simulink model "abs_pci_stress"  (Simulink 8.0)
settings: Solver=ode1  SolverMode=SingleTasking  StartTime=0.0  StopTime=999999  FixedStep=0.01  RelTol=1e-3  AbsTol=1e-6
undefined symbols (not defined in the file): abspositionscale, abspowerscale, abstemperaturescale, absvelocityscale, RTDAC4PCIBaseAddress
libraries: simulink_extras x2, simulink x1
settings Model: Creator=jims  LastModifiedBy=inteco  SimulationMode=external  ExtModeTrigDuration=60000  BufferReuse=off
settings DataIOCC: ExternalInput=[]  InitialState=[]  LimitDataPoints=off  MaxDataPoints=5000  SignalLoggingSaveFormat=ModelDataLogs  SaveOutput=off  SaveTime=off  SignalLoggingName=sigsOut
settings OptimizationCC: BlockReduction=off  BooleanDataType=off  OptimizeBlockIOStorage=off  BufferReuse=off  ExpressionFolding=off  FoldNonRolledExpr=off  LocalBlockOutputs=off  InitFltsAndDblsToZero=on
settings DebuggingCC: SaveWithParameterizedLinksMsg=none  SignalResolutionControl=TryResolveAllWithWarning  SolverPrmCheckMsg=none  MultiTaskDSMMsg=warning  MultiTaskCondExecSysMsg=none  IntegerOverflowMsg=none  FcnCallInpInsideContextMsg=UseLocalSettings  StrictBusMsg=None
settings HardwareCC: ProdIntDivRoundTo=Zero  ProdEndianess=LittleEndian  ProdHWDeviceType=Generic->32-bit x86 compatible
settings RTWCC: SystemTargetFile=rtwin.tlc  TemplateMakefile=rtwin.tmf  Description=Real-Time Windows Target  ProcessScript=rtwin_make_rtw_hook  IncludeERTFirstTime=on  RTWCompilerOptimization=On
settings CodeAppCC: MaxIdLength=95
settings RTWinTargetCC: TargetLibSuffix=_rtwin.lib  TargetPreCompLibLocation=E:\apps_W64\MATLAB\x64_R2012b\toolbox\rtw\targets\rtwin\lib\win64  CodeReplacementLibrary=ANSI_C  RTWinDir=E:/apps_W64/MATLAB/X64_R2~1/toolbox/rtw/targets/rtwin  TargetArch=win64

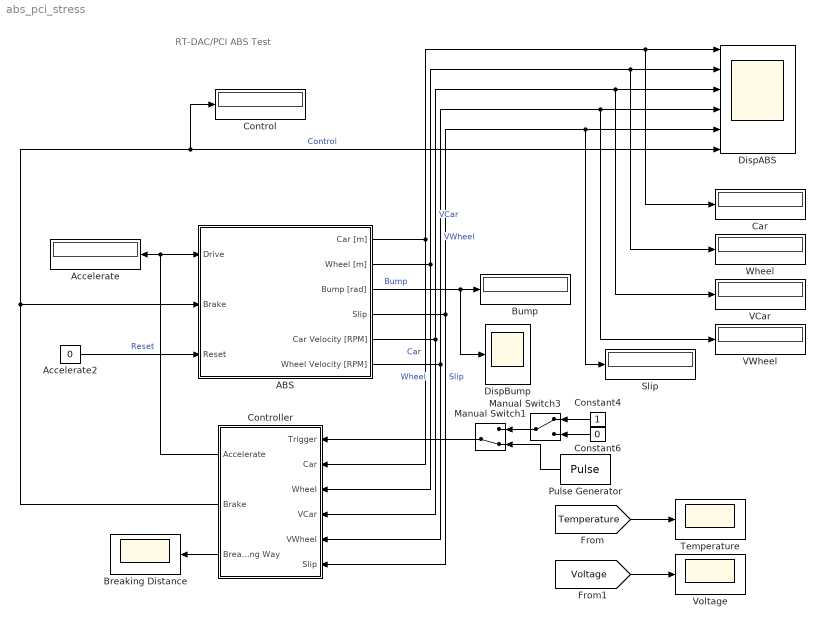
== system abs_pci_stress ==
  note: RT-DAC/PCI ABS Test
  ABS : Subsystem  mask{BaseAddress=RTDAC4PCIBaseAddress(-1,-1), T0=0.01}
      mask prompts: BaseAddress "Base Address"; T0 "Sample Time"
      mask Display: image(imread('abs.bmp'))
  Accelerate : Display
  Accelerate2 : Constant  Value=0
  Breaking Distance : Scope
      settings: TimeRange=2000  YMin=0  YMax=25  SaveName=BrakingDistance  MaxDataPoints=6000  Decimation=100
  Bump : Display
  Car : Display
  Constant4 : Constant
  Constant6 : Constant  Value=0
  Control : Display
  Controller : Subsystem
  DispABS : Scope  NumInputPorts=6
      settings: TimeRange=60  YMin=75~50~0~0~-0.4~0  YMax=250~225~1750~1750~1~1  SaveName=AbsHistory  MaxDataPoints=6000
  DispBump : Scope
      settings: TimeRange=60  YMin=3075  YMax=3275  SaveName=Vel  MaxDataPoints=6000
  Manual Switch1 : ManualSwitch  CurrentSetting=0
  Manual Switch3 : ManualSwitch
  Pulse Generator : DiscretePulseGenerator  PulseType=Time based  Period=15  PulseWidth=99
  Slip : Display
  Temperature : Scope
      settings: TimeRange=2000  YMin=20  YMax=28  SaveName=Temperature  MaxDataPoints=6000  Decimation=100
  VCar : Display
  VWheel : Display
  Voltage : Scope
      settings: TimeRange=60  YMin=18  YMax=28  SaveName=Temperature1  MaxDataPoints=6000
  Wheel : Display
  wires:
  ABS/4(Slip) -> Controller/6(Slip), DispABS/5, Slip/1  "Slip"
  ABS/6(Wheel Velocity [RPM]) -> Controller/5(VWheel), DispABS/4, VWheel/1  "VWheel"
  ABS/2(Wheel [m]) -> Controller/3(Wheel), DispABS/2, Wheel/1  "Wheel"
  ABS/1(Car [m]) -> Controller/2(Car), DispABS/1, Car/1  "Car"
  Controller/3(Breaking Way) -> Breaking Distance/1
  Constant6/1 -> Manual Switch3/2
  Constant4/1 -> Manual Switch3/1
  Controller/2(Brake) -> DispABS/6, Control/1, ABS/2(Brake)  "Control"
  ABS/5(Car Velocity [RPM]) -> Controller/4(VCar), DispABS/3, VCar/1  "VCar"
  Accelerate2/1 -> ABS/3(Reset)  "Reset"
  ABS/3(Bump [rad]) -> Bump/1, DispBump/1  "Bump"
  Controller/1(Accelerate) -> Accelerate/1, ABS/1(Drive)
  Manual Switch3/1 -> Manual Switch1/1
  Pulse Generator/1 -> Manual Switch1/2
  Manual Switch1/1 -> Controller/1(Trigger)
  [Temperature] -> Temperature/1
  [Voltage] -> Voltage/1

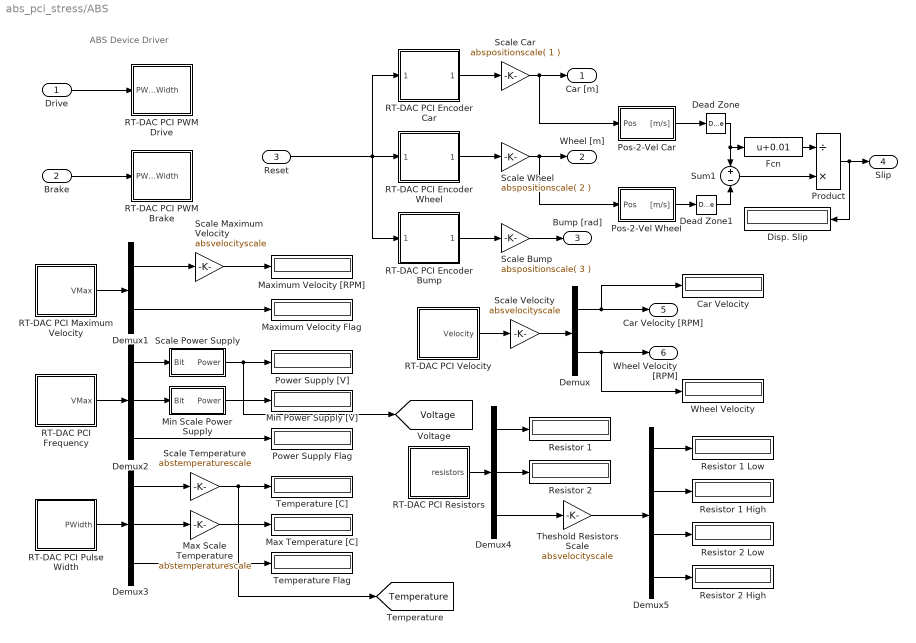
== system abs_pci_stress/ABS ==
  note: ABS Device Driver
  Drive : Inport
  Brake : Inport  Port=2
  Reset : Inport  Port=3
  Car Velocity : Display
  Dead Zone : DeadZone  LowerValue=-0.05  UpperValue=0.05  SaturateOnIntegerOverflow=on
  Dead Zone1 : DeadZone  LowerValue=-0.05  UpperValue=0.05  SaturateOnIntegerOverflow=on
  Demux : Demux  Outputs=2
  Demux1 : Demux  Outputs=2
  Demux2 : Demux  Outputs=3
  Demux3 : Demux  Outputs=3
  Demux4 : Demux  Outputs=[1 1 4]
  Demux5 : Demux
  Disp. Slip : Display
      settings: Format=bank
  Fcn : Fcn  Expr=u+0.01
  Max Scale Temperature : Gain  Gain=abstemperaturescale  OutDataTypeStr=Inherit: Same as input  ParamDataTypeStr=Inherit: Same as input
  Max Temperature [C] : Display
  Maximum Velocity Flag : Display
  Maximum Velocity [RPM] : Display
  Min Power Supply [V] : Display
  Min Scale Power Supply : Subsystem
  Pos-2-Vel Car : Subsystem
  Pos-2-Vel Wheel : Subsystem
  Power Supply Flag : Display
  Power Supply [V] : Display
  Product : Product  Inputs=/*  SaturateOnIntegerOverflow=on  InputSameDT=on  OutDataTypeStr=Inherit: Same as first input
  RT-DAC PCI Encoder Bump : Subsystem  mask(Incremental Encoders){BaseAddress=BaseAddress, ChannelIdx=2, T0=T0}
      mask prompts: BaseAddress "Base Address:"; ChannelIdx "Channel:"; T0 "Sample Time (sec):"
      mask help: RT-DAC PCI Device Driver
      mask Help: Set up each field for your specific hardware configuration.
      mask TypeOptions ChannelIdx: 0 | 1 | 2 | 3
      mask Display: plot(0,0,100,100,[90,80,80,11,11],[90,90,20,20,80],[11,80],[80,80],[80,80],[20,14],[80,85,85,80],[45,45,66,66],[45,45,74,74],[20,13,13,20],[15,27,27,15,15],[75,75,26,26,75],[33,48,48,33,33],[75,75,55,55,75],[55,55,71,71,55],[55,75,75,55,55],[33,41,41,33,33],[50,50,27,27,50],[48,56,56,48,48],[50,50,27,27,50],[62,70,70,62,62],[50,50,27,27,50])
  RT-DAC PCI Encoder Car : Subsystem  mask(Incremental Encoders){BaseAddress=BaseAddress, ChannelIdx=0, T0=T0}
      mask prompts: BaseAddress "Base Address:"; ChannelIdx "Channel:"; T0 "Sample Time (sec):"
      mask help: RT-DAC PCI Device Driver
      mask Help: Set up each field for your specific hardware configuration.
      mask TypeOptions ChannelIdx: 0 | 1 | 2 | 3
      mask Display: plot(0,0,100,100,[90,80,80,11,11],[90,90,20,20,80],[11,80],[80,80],[80,80],[20,14],[80,85,85,80],[45,45,66,66],[45,45,74,74],[20,13,13,20],[15,27,27,15,15],[75,75,26,26,75],[33,48,48,33,33],[75,75,55,55,75],[55,55,71,71,55],[55,75,75,55,55],[33,41,41,33,33],[50,50,27,27,50],[48,56,56,48,48],[50,50,27,27,50],[62,70,70,62,62],[50,50,27,27,50])
  RT-DAC PCI Encoder Wheel : Subsystem  mask(Incremental Encoders){BaseAddress=BaseAddress, ChannelIdx=1, T0=T0}
      mask prompts: BaseAddress "Base Address:"; ChannelIdx "Channel:"; T0 "Sample Time (sec):"
      mask help: RT-DAC PCI Device Driver
      mask Help: Set up each field for your specific hardware configuration.
      mask TypeOptions ChannelIdx: 0 | 1 | 2 | 3
      mask Display: plot(0,0,100,100,[90,80,80,11,11],[90,90,20,20,80],[11,80],[80,80],[80,80],[20,14],[80,85,85,80],[45,45,66,66],[45,45,74,74],[20,13,13,20],[15,27,27,15,15],[75,75,26,26,75],[33,48,48,33,33],[75,75,55,55,75],[55,55,71,71,55],[55,75,75,55,55],[33,41,41,33,33],[50,50,27,27,50],[48,56,56,48,48],[50,50,27,27,50],[62,70,70,62,62],[50,50,27,27,50])
  RT-DAC PCI Frequency : Subsystem  mask(Incremental Encoders){BaseAddress=BaseAddress, T0=T0}
      mask prompts: BaseAddress "Base Address:"; T0 "Sample Time (sec):"
      mask help: RT-DAC PCI Device Driver
      mask Help: Set up each field for your specific hardware configuration.
      mask Display: plot(0,0,100,100,[90,80,80,11,11],[90,90,20,20,80],[11,80],[80,80],[80,80],[20,14],[80,85,85,80],[45,45,66,66],[45,45,74,74],[20,13,13,20],[15,27,27,15,15],[75,75,26,26,75],[33,48,48,33,33],[75,75,55,55,75],[55,55,71,71,55],[55,75,75,55,55],[33,41,41,33,33],[50,50,27,27,50],[48,56,56,48,48],[50,50,27,27,50],[62,70,70,62,62],[50,50,27,27,50])
  RT-DAC PCI Maximum Velocity : Subsystem  mask(Incremental Encoders){BaseAddress=BaseAddress, T0=T0}
      mask prompts: BaseAddress "Base Address:"; T0 "Sample Time (sec):"
      mask help: RT-DAC PCI Device Driver
      mask Help: Set up each field for your specific hardware configuration.
      mask Display: plot(0,0,100,100,[90,80,80,11,11],[90,90,20,20,80],[11,80],[80,80],[80,80],[20,14],[80,85,85,80],[45,45,66,66],[45,45,74,74],[20,13,13,20],[15,27,27,15,15],[75,75,26,26,75],[33,48,48,33,33],[75,75,55,55,75],[55,55,71,71,55],[55,75,75,55,55],[33,41,41,33,33],[50,50,27,27,50],[48,56,56,48,48],[50,50,27,27,50],[62,70,70,62,62],[50,50,27,27,50])
  RT-DAC PCI PWM Brake : Subsystem  mask(PWM Module){BaseAddress=BaseAddress, ChanIdx=1, ChanMode=8 Bit, ChanPresc=7, SetOutputsFlag=on, SetOutputsValue=0, T0=T0}
      mask prompts: BaseAddress "IO Base Address:"; ChanIdx "Channel:"; ChanMode "Channel Mode:"; ChanPresc "Channel Prescaler:"; SetOutputsFlag "Set Outputs At Termination"; SetOutputsValue "Termination Outputs:"; T0 "Sample Time (sec):"
      mask help: RT-DAC PCI Device Driver
      mask Help: Set up each field for your specific hardware configuration.
      mask TypeOptions ChanIdx: 0 | 1 | 2 | 3
      mask TypeOptions ChanMode: 8 Bit | 12 Bit
      mask Display: plot(0,0,100,100,[90,80,80,11,11],[90,90,20,20,80],[11,80],[80,80],[80,80],[20,14],[80,85,85,80],[45,45,66,66],[45,45,74,74],[20,13,13,20],[15,27,27,15,15],[75,75,26,26,75],[33,48,48,33,33],[75,75,55,55,75],[55,55,71,71,55],[55,75,75,55,55],[33,41,41,33,33],[50,50,27,27,50],[48,56,56,48,48],[50,50,27,27,50],[62,70,70,62,62],[50,50,27,27,50])
  RT-DAC PCI PWM Drive : Subsystem  mask(PWM Module){BaseAddress=BaseAddress, ChanIdx=0, ChanMode=8 Bit, ChanPresc=7, SetOutputsFlag=on, SetOutputsValue=0, T0=T0}
      mask prompts: BaseAddress "IO Base Address:"; ChanIdx "Channel:"; ChanMode "Channel Mode:"; ChanPresc "Channel Prescaler:"; SetOutputsFlag "Set Outputs At Termination"; SetOutputsValue "Termination Outputs:"; T0 "Sample Time (sec):"
      mask help: RT-DAC PCI Device Driver
      mask Help: Set up each field for your specific hardware configuration.
      mask TypeOptions ChanIdx: 0 | 1 | 2 | 3
      mask TypeOptions ChanMode: 8 Bit | 12 Bit
      mask Display: plot(0,0,100,100,[90,80,80,11,11],[90,90,20,20,80],[11,80],[80,80],[80,80],[20,14],[80,85,85,80],[45,45,66,66],[45,45,74,74],[20,13,13,20],[15,27,27,15,15],[75,75,26,26,75],[33,48,48,33,33],[75,75,55,55,75],[55,55,71,71,55],[55,75,75,55,55],[33,41,41,33,33],[50,50,27,27,50],[48,56,56,48,48],[50,50,27,27,50],[62,70,70,62,62],[50,50,27,27,50])
  RT-DAC PCI Pulse Width : Subsystem  mask(Incremental Encoders){BaseAddress=BaseAddress, T0=T0}
      mask prompts: BaseAddress "Base Address:"; T0 "Sample Time (sec):"
      mask help: RT-DAC PCI Device Driver
      mask Help: Set up each field for your specific hardware configuration.
      mask Display: plot(0,0,100,100,[90,80,80,11,11],[90,90,20,20,80],[11,80],[80,80],[80,80],[20,14],[80,85,85,80],[45,45,66,66],[45,45,74,74],[20,13,13,20],[15,27,27,15,15],[75,75,26,26,75],[33,48,48,33,33],[75,75,55,55,75],[55,55,71,71,55],[55,75,75,55,55],[33,41,41,33,33],[50,50,27,27,50],[48,56,56,48,48],[50,50,27,27,50],[62,70,70,62,62],[50,50,27,27,50])
  RT-DAC PCI Resistors : Subsystem  mask(Incremental Encoders){BaseAddress=BaseAddress, T0=T0}
      mask prompts: BaseAddress "Base Address:"; T0 "Sample Time (sec):"
      mask help: RT-DAC PCI Device Driver
      mask Help: Set up each field for your specific hardware configuration.
      mask Display: plot(0,0,100,100,[90,80,80,11,11],[90,90,20,20,80],[11,80],[80,80],[80,80],[20,14],[80,85,85,80],[45,45,66,66],[45,45,74,74],[20,13,13,20],[15,27,27,15,15],[75,75,26,26,75],[33,48,48,33,33],[75,75,55,55,75],[55,55,71,71,55],[55,75,75,55,55],[33,41,41,33,33],[50,50,27,27,50],[48,56,56,48,48],[50,50,27,27,50],[62,70,70,62,62],[50,50,27,27,50])
  RT-DAC PCI Velocity : Subsystem  mask(Incremental Encoders){BaseAddress=BaseAddress, T0=T0}
      mask prompts: BaseAddress "Base Address:"; T0 "Sample Time (sec):"
      mask help: RT-DAC PCI Device Driver
      mask Help: Set up each field for your specific hardware configuration.
      mask Display: plot(0,0,100,100,[90,80,80,11,11],[90,90,20,20,80],[11,80],[80,80],[80,80],[20,14],[80,85,85,80],[45,45,66,66],[45,45,74,74],[20,13,13,20],[15,27,27,15,15],[75,75,26,26,75],[33,48,48,33,33],[75,75,55,55,75],[55,55,71,71,55],[55,75,75,55,55],[33,41,41,33,33],[50,50,27,27,50],[48,56,56,48,48],[50,50,27,27,50],[62,70,70,62,62],[50,50,27,27,50])
  Resistor 1 : Display
  Resistor 1 High : Display
  Resistor 1 Low : Display
  Resistor 2 : Display
  Resistor 2 High : Display
  Resistor 2 Low : Display
  Scale Bump : Gain  Gain=abspositionscale( 3 )  OutDataTypeStr=Inherit: Same as input  ParamDataTypeStr=Inherit: Same as input
  Scale Car : Gain  Gain=abspositionscale( 1 )  OutDataTypeStr=Inherit: Same as input  ParamDataTypeStr=Inherit: Same as input
  Scale Maximum Velocity : Gain  Gain=absvelocityscale  OutDataTypeStr=Inherit: Same as input  ParamDataTypeStr=Inherit: Same as input
  Scale Velocity : Gain  Gain=absvelocityscale  OutDataTypeStr=Inherit: Same as input  ParamDataTypeStr=Inherit: Same as input
  Scale Wheel : Gain  Gain=abspositionscale( 2 )  OutDataTypeStr=Inherit: Same as input  ParamDataTypeStr=Inherit: Same as input
  Scale Power Supply : Subsystem
  Scale Temperature : Gain  Gain=abstemperaturescale  OutDataTypeStr=Inherit: Same as input  ParamDataTypeStr=Inherit: Same as input
  Sum1 : Sum  Inputs=+-  SaturateOnIntegerOverflow=on  InputSameDT=on  OutDataTypeStr=Inherit: Same as first input
  Temperature Flag : Display
  Temperature [C] : Display
  Theshold Resistors Scale : Gain  Gain=absvelocityscale  OutDataTypeStr=Inherit: Same as input  ParamDataTypeStr=Inherit: Same as input
  Wheel Velocity : Display
  Car [m] : Outport
  Wheel [m] : Outport  Port=2
  Bump [rad] : Outport  Port=3
  Slip : Outport  Port=4
  Car Velocity [RPM] : Outport  Port=5
  Wheel Velocity [RPM] : Outport  Port=6
  tag scope: Temperature=global, Voltage=global
  wires:
  RT-DAC PCI Encoder Car/1(Encoder Counter) -> Scale Car/1
  RT-DAC PCI Encoder Wheel/1(Encoder Counter) -> Scale Wheel/1
  RT-DAC PCI Encoder Bump/1(Encoder Counter) -> Scale Bump/1
  Scale Car/1 -> Car [m]/1, Pos-2-Vel Car/1(Pos)
  Scale Wheel/1 -> Wheel [m]/1, Pos-2-Vel Wheel/1(Pos)
  Scale Bump/1 -> Bump [rad]/1
  RT-DAC PCI Velocity/1(Velocity) -> Scale Velocity/1
  Scale Velocity/1 -> Demux/1
  Scale Power Supply/1(Power) -> Power Supply [V]/1, [Voltage]
  Scale Temperature/1 -> Temperature [C]/1, [Temperature]
  Drive/1 -> RT-DAC PCI PWM Drive/1(PWM Width)
  Brake/1 -> RT-DAC PCI PWM Brake/1(PWM Width)
  Demux/1 -> Car Velocity [RPM]/1, Car Velocity/1
  Demux/2 -> Wheel Velocity [RPM]/1, Wheel Velocity/1
  RT-DAC PCI Maximum Velocity/1(VMax) -> Demux1/1
  Demux1/1 -> Scale Maximum Velocity/1
  Scale Maximum Velocity/1 -> Maximum Velocity [RPM]/1
  Demux1/2 -> Maximum Velocity Flag/1
  RT-DAC PCI Frequency/1(VMax) -> Demux2/1
  Demux2/1 -> Scale Power Supply/1(Bit)
  RT-DAC PCI Pulse Width/1(PWidth) -> Demux3/1
  Demux3/1 -> Scale Temperature/1
  Reset/1 -> RT-DAC PCI Encoder Wheel/1(Reset), RT-DAC PCI Encoder Car/1(Reset), RT-DAC PCI Encoder Bump/1(Reset)
  Demux2/2 -> Min Scale Power Supply/1(Bit)
  Min Scale Power Supply/1(Power) -> Min Power Supply [V]/1
  Demux2/3 -> Power Supply Flag/1
  Max Scale Temperature/1 -> Max Temperature [C]/1
  Demux3/2 -> Max Scale Temperature/1
  Demux3/3 -> Temperature Flag/1
  RT-DAC PCI Resistors/1(resistors) -> Demux4/1
  Demux4/1 -> Resistor 1/1
  Demux4/2 -> Resistor 2/1
  Demux4/3 -> Theshold Resistors Scale/1
  Theshold Resistors Scale/1 -> Demux5/1
  Demux5/1 -> Resistor 1 Low/1
  Demux5/2 -> Resistor 1 High/1
  Demux5/3 -> Resistor 2 Low/1
  Demux5/4 -> Resistor 2 High/1
  Sum1/1 -> Product/2
  Fcn/1 -> Product/1
  Product/1 -> Slip/1, Disp. Slip/1
  Pos-2-Vel Wheel/1("[m/s]") -> Dead Zone1/1
  Pos-2-Vel Car/1("[m/s]") -> Dead Zone/1
  Dead Zone/1 -> Sum1/1, Fcn/1
  Dead Zone1/1 -> Sum1/2

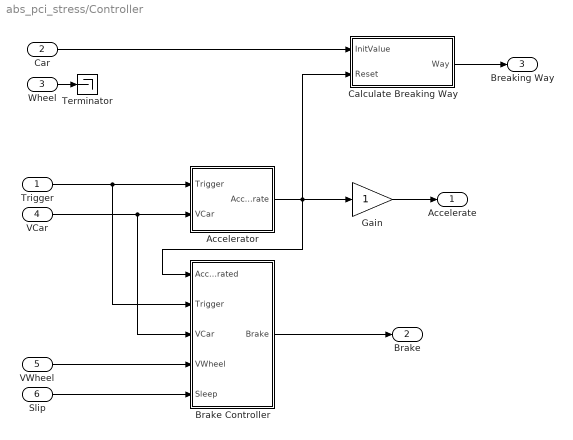
== system abs_pci_stress/Controller ==
  Trigger : Inport
  Car : Inport  Port=2
  Wheel : Inport  Port=3
  VCar : Inport  Port=4
  VWheel : Inport  Port=5
  Slip : Inport  Port=6
  Accelerator : Subsystem
  Brake Controller : Subsystem
  Calculate Breaking Way : Subsystem
  Gain : Gain  SaturateOnIntegerOverflow=on  OutDataTypeStr=Inherit: Same as input  ParamDataTypeStr=Inherit: Same as input
  Terminator : Terminator
  Accelerate : Outport
  Brake : Outport  Port=2
  Breaking Way : Outport  Port=3
  wires:
  Trigger/1 -> Accelerator/1(Trigger), Brake Controller/2(Trigger)
  Calculate Breaking Way/1(Way) -> Breaking Way/1
  VCar/1 -> Brake Controller/3(VCar), Accelerator/2(VCar)
  Car/1 -> Calculate Breaking Way/1(InitValue)
  Slip/1 -> Brake Controller/5(Sleep)
  Accelerator/1(Accelerate) -> Calculate Breaking Way/2(Reset), Brake Controller/1(Accelerated), Gain/1
  VWheel/1 -> Brake Controller/4(VWheel)
  Brake Controller/1(Brake) -> Brake/1
  Wheel/1 -> Terminator/1
  Gain/1 -> Accelerate/1

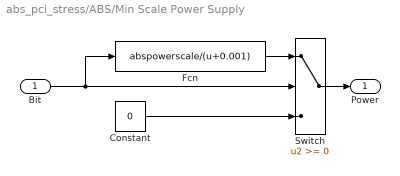
== system abs_pci_stress/ABS/Min Scale Power Supply ==
  Bit : Inport
  Constant : Constant  Value=0
  Fcn : Fcn  Expr=abspowerscale/(u+0.001)
  Switch : Switch  SaturateOnIntegerOverflow=on  InputSameDT=on
  Power : Outport
  wires:
  Constant/1 -> Switch/3
  Fcn/1 -> Switch/1
  Switch/1 -> Power/1
  Bit/1 -> Fcn/1, Switch/2

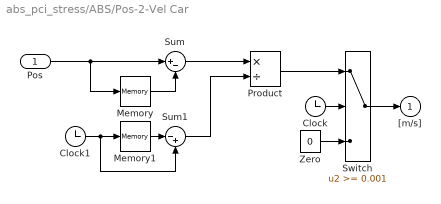
== system abs_pci_stress/ABS/Pos-2-Vel Car ==
  Pos : Inport
  Clock : Clock
  Clock1 : Clock
  Memory : Memory  InheritSampleTime=on
  Memory1 : Memory  InheritSampleTime=on
  Product : Product  Inputs=*/  SaturateOnIntegerOverflow=on  InputSameDT=on  OutDataTypeStr=Inherit: Same as first input
  Sum : Sum  Inputs=|+-  SaturateOnIntegerOverflow=on  InputSameDT=on  OutDataTypeStr=Inherit: Same as first input
  Sum1 : Sum  Inputs=|-+  SaturateOnIntegerOverflow=on  InputSameDT=on  OutDataTypeStr=Inherit: Same as first input
  Switch : Switch  Threshold=0.001  SaturateOnIntegerOverflow=on  InputSameDT=on
  Zero : Constant  Value=0
  "[m/s]" : Outport
  wires:
  Sum1/1 -> Product/2
  Memory1/1 -> Sum1/1
  Clock1/1 -> Sum1/2, Memory1/1
  Sum/1 -> Product/1
  Product/1 -> Switch/1
  Zero/1 -> Switch/3
  Switch/1 -> "[m/s]"/1
  Clock/1 -> Switch/2
  Memory/1 -> Sum/2
  Pos/1 -> Sum/1, Memory/1

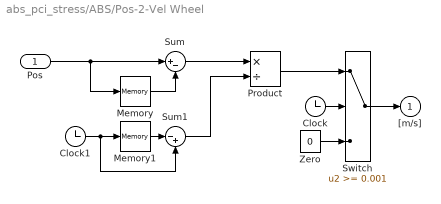
== system abs_pci_stress/ABS/Pos-2-Vel Wheel ==
  Pos : Inport
  Clock : Clock
  Clock1 : Clock
  Memory : Memory  InheritSampleTime=on
  Memory1 : Memory  InheritSampleTime=on
  Product : Product  Inputs=*/  SaturateOnIntegerOverflow=on  InputSameDT=on  OutDataTypeStr=Inherit: Same as first input
  Sum : Sum  Inputs=|+-  SaturateOnIntegerOverflow=on  InputSameDT=on  OutDataTypeStr=Inherit: Same as first input
  Sum1 : Sum  Inputs=|-+  SaturateOnIntegerOverflow=on  InputSameDT=on  OutDataTypeStr=Inherit: Same as first input
  Switch : Switch  Threshold=0.001  SaturateOnIntegerOverflow=on  InputSameDT=on
  Zero : Constant  Value=0
  "[m/s]" : Outport
  wires:
  Pos/1 -> Memory/1, Sum/1
  Memory/1 -> Sum/2
  Clock/1 -> Switch/2
  Switch/1 -> "[m/s]"/1
  Zero/1 -> Switch/3
  Product/1 -> Switch/1
  Sum/1 -> Product/1
  Clock1/1 -> Memory1/1, Sum1/2
  Memory1/1 -> Sum1/1
  Sum1/1 -> Product/2

== system abs_pci_stress/ABS/RT-DAC PCI Encoder Bump ==
  Reset : Inport
  RT-DAC PCI Encoder : S-Function  FunctionName=rtdacpci_abs_encoder  Parameters=BaseAddress, ChannelIdx, T0  EnableBusSupport=off
  Encoder Counter : Outport
  wires:
  Reset/1 -> RT-DAC PCI Encoder/1
  RT-DAC PCI Encoder/1 -> Encoder Counter/1

== system abs_pci_stress/ABS/RT-DAC PCI Encoder Car ==
  Reset : Inport
  RT-DAC PCI Encoder : S-Function  FunctionName=rtdacpci_abs_encoder  Parameters=BaseAddress, ChannelIdx, T0  EnableBusSupport=off
  Encoder Counter : Outport
  wires:
  Reset/1 -> RT-DAC PCI Encoder/1
  RT-DAC PCI Encoder/1 -> Encoder Counter/1

== system abs_pci_stress/ABS/RT-DAC PCI Encoder Wheel ==
  Reset : Inport
  RT-DAC PCI Encoder : S-Function  FunctionName=rtdacpci_abs_encoder  Parameters=BaseAddress, ChannelIdx, T0  EnableBusSupport=off
  Encoder Counter : Outport
  wires:
  RT-DAC PCI Encoder/1 -> Encoder Counter/1
  Reset/1 -> RT-DAC PCI Encoder/1

== system abs_pci_stress/ABS/RT-DAC PCI Frequency ==
  RT-DAC PCI Frequency : S-Function  FunctionName=rtdacpci_abs_frequency  Parameters=BaseAddress, T0  EnableBusSupport=off
  VMax : Outport
  wires:
  RT-DAC PCI Frequency/1 -> VMax/1

== system abs_pci_stress/ABS/RT-DAC PCI Maximum Velocity ==
  RT-DAC PCI VMax : S-Function  FunctionName=rtdacpci_abs_vmax  Parameters=BaseAddress, T0  EnableBusSupport=off
  VMax : Outport
  wires:
  RT-DAC PCI VMax/1 -> VMax/1

== system abs_pci_stress/ABS/RT-DAC PCI PWM Brake ==
  PWM Width : Inport
  "RT-DAC PCI PWM " : S-Function  FunctionName=rtdacpci_abs_pwm  Parameters=BaseAddress, ChanIdx, ChanMode, ChanPresc, SetOutputsFlag, SetOutputsValue, T0  EnableBusSupport=off
  wires:
  PWM Width/1 -> "RT-DAC PCI PWM "/1

== system abs_pci_stress/ABS/RT-DAC PCI PWM Drive ==
  PWM Width : Inport
  "RT-DAC PCI PWM " : S-Function  FunctionName=rtdacpci_abs_pwm  Parameters=BaseAddress, ChanIdx, ChanMode, ChanPresc, SetOutputsFlag, SetOutputsValue, T0  EnableBusSupport=off
  wires:
  PWM Width/1 -> "RT-DAC PCI PWM "/1

== system abs_pci_stress/ABS/RT-DAC PCI Pulse Width ==
  RT-DAC PCI Pulse Width : S-Function  FunctionName=rtdacpci_abs_pulsewidth  Parameters=BaseAddress, T0  EnableBusSupport=off
  PWidth : Outport
  wires:
  RT-DAC PCI Pulse Width/1 -> PWidth/1

== system abs_pci_stress/ABS/RT-DAC PCI Resistors ==
  RT-DAC PCI Resistors : S-Function  FunctionName=rtdacpci_abs_resistors  Parameters=BaseAddress, T0  EnableBusSupport=off
  resistors : Outport
  wires:
  RT-DAC PCI Resistors/1 -> resistors/1

== system abs_pci_stress/ABS/RT-DAC PCI Velocity ==
  RT-DAC PCI Velocity : S-Function  FunctionName=rtdacpci_abs_velocity  Parameters=BaseAddress, T0  EnableBusSupport=off
  Velocity : Outport
  wires:
  RT-DAC PCI Velocity/1 -> Velocity/1

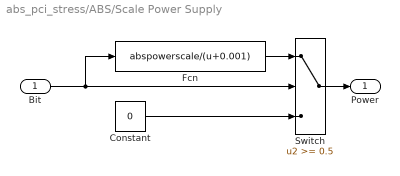
== system abs_pci_stress/ABS/Scale Power Supply ==
  Bit : Inport
  Constant : Constant  Value=0
  Fcn : Fcn  Expr=abspowerscale/(u+0.001)
  Switch : Switch  Threshold=0.5  SaturateOnIntegerOverflow=on  InputSameDT=on
  Power : Outport
  wires:
  Bit/1 -> Switch/2, Fcn/1
  Switch/1 -> Power/1
  Fcn/1 -> Switch/1
  Constant/1 -> Switch/3

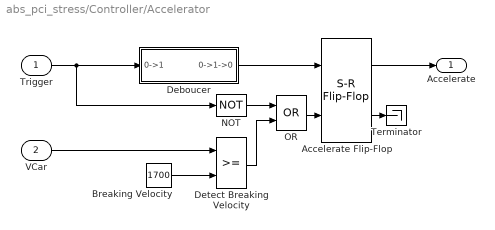
== system abs_pci_stress/Controller/Accelerator ==
  Trigger : Inport
  VCar : Inport  Port=2
  Accelerate Flip-Flop : simulink_extras/Flip Flops/S-R Flip-Flop  initial_condition=0
  Breaking Velocity : Constant  Value=1700
  Deboucer : Subsystem
  Detect Breaking Velocity : RelationalOperator  InputSameDT=on
  NOT : Logic  Operator=NOT
  OR : Logic  Operator=OR
  Terminator : Terminator
  Accelerate : Outport
  wires:
  Deboucer/1(0->1->0) -> Accelerate Flip-Flop/1
  Breaking Velocity/1 -> Detect Breaking Velocity/2
  OR/1 -> Accelerate Flip-Flop/2
  Detect Breaking Velocity/1 -> OR/2
  NOT/1 -> OR/1
  Accelerate Flip-Flop/2 -> Terminator/1
  Trigger/1 -> Deboucer/1(0->1), NOT/1
  VCar/1 -> Detect Breaking Velocity/1
  Accelerate Flip-Flop/1 -> Accelerate/1

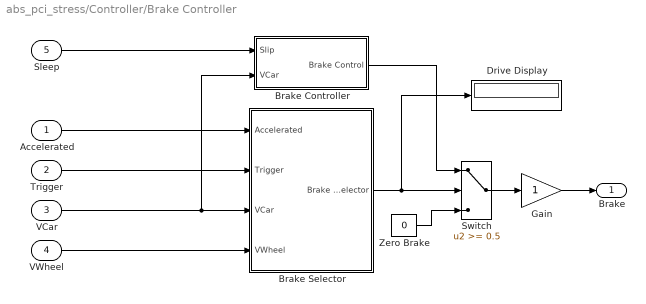
== system abs_pci_stress/Controller/Brake Controller ==
  Accelerated : Inport
  Trigger : Inport  Port=2
  VCar : Inport  Port=3
  VWheel : Inport  Port=4
  Sleep : Inport  Port=5
  Brake Controller : Subsystem
  Brake Selector : Subsystem
  Drive Display : Display
  Gain : Gain  SaturateOnIntegerOverflow=on  OutDataTypeStr=Inherit: Same as input  ParamDataTypeStr=Inherit: Same as input
  Switch : Switch  Threshold=0.5  InputSameDT=on
  Zero Brake : Constant  Value=0
  Brake : Outport
  wires:
  Accelerated/1 -> Brake Selector/1(Accelerated)
  Trigger/1 -> Brake Selector/2(Trigger)
  VCar/1 -> Brake Selector/3(VCar), Brake Controller/2(VCar)
  VWheel/1 -> Brake Selector/4(VWheel)
  Switch/1 -> Gain/1
  Brake Selector/1(Brake Selector) -> Switch/2, Drive Display/1
  Zero Brake/1 -> Switch/3
  Sleep/1 -> Brake Controller/1(Slip)
  Brake Controller/1(Brake Control) -> Switch/1
  Gain/1 -> Brake/1

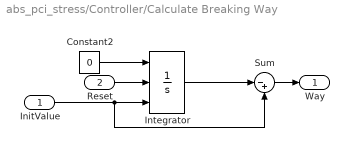
== system abs_pci_stress/Controller/Calculate Breaking Way ==
  InitValue : Inport
  Reset : Inport  Port=2
  Constant2 : Constant  Value=0
  Integrator : Integrator  ExternalReset=level  InitialConditionSource=external
  Sum : Sum  Inputs=|-+  SaturateOnIntegerOverflow=on  InputSameDT=on  OutDataTypeStr=Inherit: Same as first input
  Way : Outport
  wires:
  Constant2/1 -> Integrator/1
  Integrator/1 -> Sum/1
  InitValue/1 -> Sum/2, Integrator/3
  Reset/1 -> Integrator/2
  Sum/1 -> Way/1

== system abs_pci_stress/Controller/Accelerator/Deboucer ==
  0->1 : Inport
  AND : Logic
  Memory : Memory
  NOT : Logic  Operator=NOT
  0->1->0 : Outport
  wires:
  NOT/1 -> AND/1
  Memory/1 -> NOT/1
  0->1/1 -> AND/2, Memory/1
  AND/1 -> 0->1->0/1

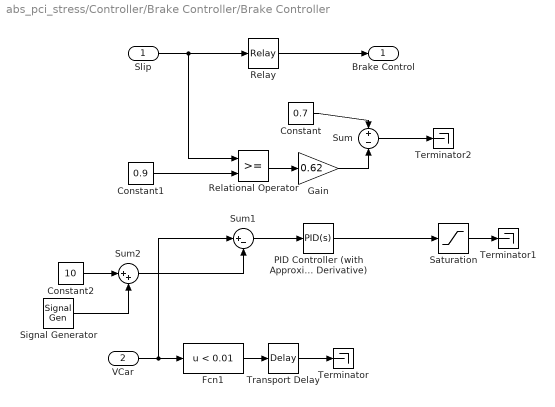
== system abs_pci_stress/Controller/Brake Controller/Brake Controller ==
  Slip : Inport
  VCar : Inport  Port=2
  Constant : Constant  Value=0.7
  Constant1 : Constant  Value=0.9
  Constant2 : Constant  Value=10
  Fcn1 : Fcn  Expr=u < 0.01
  Gain : Gain  Gain=0.62  SaturateOnIntegerOverflow=on  OutDataTypeStr=Inherit: Same as input  ParamDataTypeStr=Inherit: Same as input
  PID Controller (with Approximate Derivative) : simulink/Continuous/PID Controller  Controller=PID  TimeDomain=Continuous-time  SampleTime=1  IntegratorMethod=Forward Euler  FilterMethod=Forward Euler  Form=Parallel  P=0.2  I=0  D=0  N=100  InitialConditionSource=internal  InitialConditionForIntegrator=0  InitialConditionForFilter=0  ExternalReset=none  LimitOutput=off  UpperSaturationLimit=inf  LowerSaturationLimit=-inf  LinearizeAsGain=off  AntiWindupMode=none  Kb=1  TrackingMode=off  Kt=1  PParamMin=[]  PParamMax=[]  IParamMin=[]  IParamMax=[]  DParamMin=[]  DParamMax=[]  NParamMin=[]  NParamMax=[]  KbParamMin=[]  KbParamMax=[]  KtParamMin=[]  KtParamMax=[]  POutMin=[]  POutMax=[]  IOutMin=[]  IOutMax=[]  DOutMin=[]  DOutMax=[]  NOutMin=[]  NOutMax=[]  KbOutMin=[]  KbOutMax=[]  KtOutMin=[]  KtOutMax=[]  IntegratorOutMin=[]  IntegratorOutMax=[]  FilterOutMin=[]  FilterOutMax=[]  SumOutMin=[]  SumOutMax=[]  SumI1OutMin=[]  SumI1OutMax=[]  SumI2OutMin=[]  SumI2OutMax=[]  SumI3OutMin=[]  SumI3OutMax=[]  SumDOutMin=[]  SumDOutMax=[]  SaturationOutMin=[]  SaturationOutMax=[]  IntegratorContinuousStateAttributes=''  IntegratorStateMustResolveToSignalObject=off  IntegratorRTWStateStorageClass=Auto  FilterContinuousStateAttributes=''  FilterStateMustResolveToSignalObject=off  FilterRTWStateStorageClass=Auto
  Relational Operator : RelationalOperator  InputSameDT=on
  Relay : Relay  OnSwitchValue=0.3  OffSwitchValue=0.3  OnOutputValue=0  OffOutputValue=0.4
  Saturation : Saturate  UpperLimit=0.7  LowerLimit=0
  Signal Generator : SignalGenerator  WaveForm=square  Amplitude=2  Frequency=0.03
  Sum : Sum  Inputs=+-  SaturateOnIntegerOverflow=on  InputSameDT=on  OutDataTypeStr=Inherit: Same as first input
  Sum1 : Sum  Inputs=|+-  SaturateOnIntegerOverflow=on  InputSameDT=on  OutDataTypeStr=Inherit: Same as first input
  Sum2 : Sum  Inputs=|++  SaturateOnIntegerOverflow=on  InputSameDT=on  OutDataTypeStr=Inherit: Same as first input
  Terminator : Terminator
  Terminator1 : Terminator
  Terminator2 : Terminator
  Transport Delay : TransportDelay  DelayTime=0.5  FixedBuffer=on
  Brake Control : Outport
  wires:
  Relay/1 -> Brake Control/1
  Signal Generator/1 -> Sum2/2
  Constant2/1 -> Sum2/1
  Sum2/1 -> Sum1/2
  PID Controller (with Approximate Derivative)/1 -> Saturation/1
  Sum1/1 -> PID Controller (with Approximate Derivative)/1
  Gain/1 -> Sum/2
  Constant/1 -> Sum/1
  Constant1/1 -> Relational Operator/2
  Relational Operator/1 -> Gain/1
  VCar/1 -> Sum1/1, Fcn1/1
  Fcn1/1 -> Transport Delay/1
  Slip/1 -> Relay/1, Relational Operator/1
  Sum/1 -> Terminator2/1
  Saturation/1 -> Terminator1/1
  Transport Delay/1 -> Terminator/1

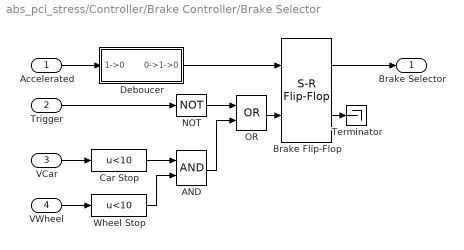
== system abs_pci_stress/Controller/Brake Controller/Brake Selector ==
  Accelerated : Inport
  Trigger : Inport  Port=2
  VCar : Inport  Port=3
  VWheel : Inport  Port=4
  AND : Logic
  Brake Flip-Flop : simulink_extras/Flip Flops/S-R Flip-Flop  initial_condition=0
  Car Stop : Fcn  Expr=u<10
  Deboucer : Subsystem
  NOT : Logic  Operator=NOT
  OR : Logic  Operator=OR
  Terminator : Terminator
  Wheel Stop : Fcn  Expr=u<10
  Brake Selector : Outport
  wires:
  Brake Flip-Flop/2 -> Terminator/1
  NOT/1 -> OR/1
  AND/1 -> OR/2
  OR/1 -> Brake Flip-Flop/2
  Deboucer/1(0->1->0) -> Brake Flip-Flop/1
  Car Stop/1 -> AND/1
  Wheel Stop/1 -> AND/2
  Brake Flip-Flop/1 -> Brake Selector/1
  Accelerated/1 -> Deboucer/1(1->0)
  Trigger/1 -> NOT/1
  VCar/1 -> Car Stop/1
  VWheel/1 -> Wheel Stop/1

== system abs_pci_stress/Controller/Brake Controller/Brake Selector/Deboucer ==
  1->0 : Inport
  AND : Logic
  Memory : Memory
  NOT : Logic  Operator=NOT
  0->1->0 : Outport
  wires:
  AND/1 -> 0->1->0/1
  1->0/1 -> Memory/1, NOT/1
  Memory/1 -> AND/1
  NOT/1 -> AND/2
